simulink model "modeling"  (R2016a)
settings: Solver=VariableStepAuto  StartTime=0.0  StopTime=10.0  RelTol=1e-3
settings Model: Creator=USER  LastModifiedBy=USER

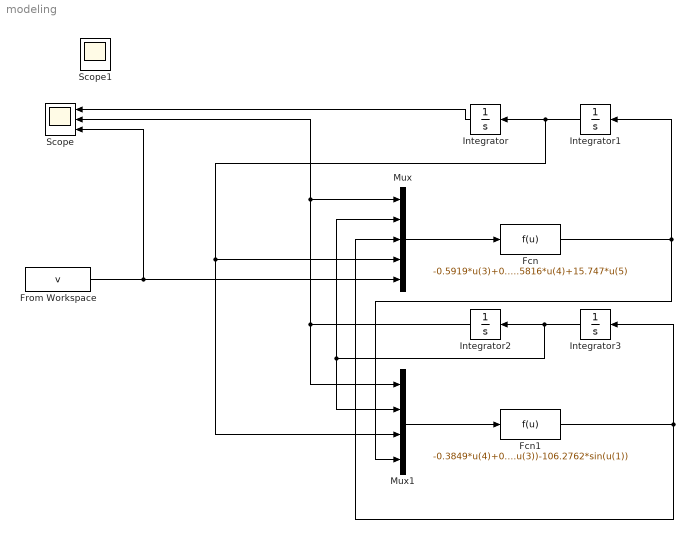
== system modeling ==
  Fcn : Fcn  Expr=-0.5919*u(3)+0.3735*(2*cos(u(1))*u(3)-sin(2*u(1))/cos(u(1))*u(2))+6.4125*u(2)-140.5816*u(4)+15.747*u(5)
  Fcn1 : Fcn  Expr=-0.3849*u(4)+0.8639*cos(u(1))*u(4)-1.2506*(u(2)+u(3))-106.2762*sin(u(1))
  From Workspace : FromWorkspace  VariableName=v  SampleTime=0
  Integrator{,1..3} (4 alike) : Integrator
  Mux : Mux  Inputs=5
  Mux1 : Mux
  Scope : Scope  NumInputPorts=3
  Scope1 : Scope
  wires:
  Integrator1/1 -> Mux1/3, Mux/4, Integrator/1
  Integrator3/1 -> Mux/2, Mux1/2, Integrator2/1
  Integrator/1 -> Scope/1
  Integrator2/1 -> Scope/2, Mux/1, Mux1/1
  Mux1/1 -> Fcn1/1
  Mux/1 -> Fcn/1
  Fcn1/1 -> Integrator3/1, Mux/3
  Fcn/1 -> Mux1/4, Integrator1/1
  From Workspace/1 -> Scope/3, Mux/5
